simulink model "Ammonia_Model"  (R2023a)
settings: Solver=FixedStepAuto  StartTime=0.0  StopTime=Z  FixedStep=1/24  RelTol=1e-3
values from neighbouring files (symbols this model uses):
  c_eh = 0.85    [Model_Parameters.m]
  cc_AH2_l = 0.6    [Model_Parameters.m]
  cc_AH2_r = 0.75    [Model_Parameters.m]
  cc_AH2_z = 0.65    [Model_Parameters.m]
  cc_e = -0.85    [Model_Parameters.m]
  id_l_A = id_l*id_frac_A    (= 0.0480384)    [Model_Parameters.m]
  id_r_A = id_r*id_frac_A    (= 0.1479168)    [Model_Parameters.m]
  id_z_A = id_z*id_frac_A    (= 0.114048)    [Model_Parameters.m]
  R_ammonia = 0.025    [Model_Parameters.m]
  R_H2 = 0.05    [Model_Parameters.m]
  R_lh = 0.025    [Model_Parameters.m]
  R_ng = 0.025    [Model_Parameters.m]
  S_a_l = 0.3    [Model_Parameters.m]
  S_a_r = 0.2    [Model_Parameters.m]
  S_a_z = 0.25    [Model_Parameters.m]
libraries: fl_lib x72, nesl_utility x50, ee_lib x27
(part 1 of 2)
settings Model: Creator=pienv  LastModifiedBy=pienv

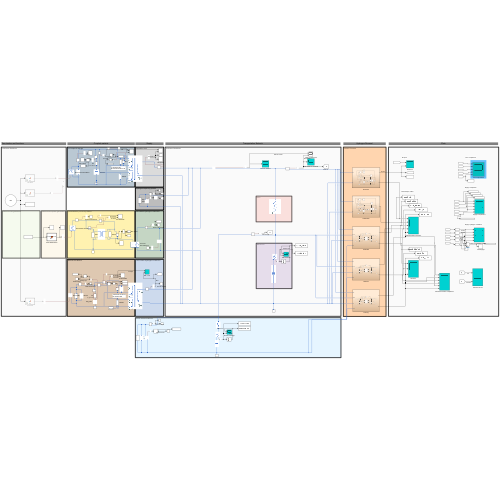
[thumbnail: Simulink's stored preview of the top-level diagram]
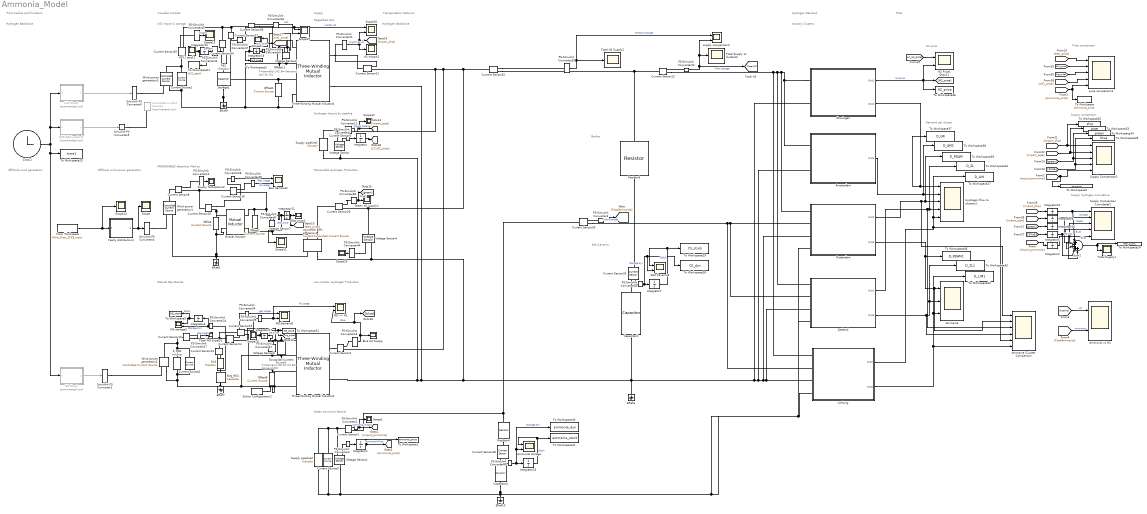
== system Ammonia_Model ==
  note: Supply hydrogen cumulative
  note: T=demand NG for H2
      | B= demand NG
  note: Demand per cluster
  note: LH2 Import & storage
  note: Plots
  note: Salt Caverns
  note: Offshore wind generation
  note: Price comparison
  note: Broker
  note: Coupled markets
  note: Natural Gas Market
  note: (RENEWABLE) electricity Market
  note: Hydrogen Backbone
  note: Hydrogen Import by pipeline
  note: Offshore wind power generation
  note: Green ammonia Market
  note: Time tracker and functions
  note: T=demand LH2
      | B= demand LH2 for H2
  note: H2 price
  note: Supply
  note: Hydrogen Demand
  note: Regasified LH2
  note: Renewable Hydrogen Production
  note: Transportation Network
  note: Hydrogen Backbone
  note: Industry Clusters
  note: Supply comparison
  note: Low-Carbon Hydrogen Production
  Ammonia : Scope  NumInputPorts=3
  Ammonia CLuster Comparison : Scope  NumInputPorts=6
  Ammonia storage : Scope  NumInputPorts=2
  Ammonia vs H2 : Scope  NumInputPorts=2
  Amsterdam : Subsystem
  Blue H2 Supply : Scope
  Capacitor3 : fl_lib/Electrical/Electrical Elements/Capacitor  c=C_sc F  r=0 Ohm  g=0 1/Ohm  i_specify=on  i_priority=None  i=0.1 A  i_nominal_specify=off  i_nominal_unit=A  i_nominal_value=0.1  v_specify=off  v_priority=None  v=0 V  v_nominal_specify=off  v_nominal_unit=V  v_nominal_value=1  vc_specify=off  vc_priority=High  vc=0 V  vc_nominal_specify=off  vc_nominal_unit=V  vc_nominal_value=1
  Capacitor4 : fl_lib/Electrical/Electrical Elements/Capacitor  c=C_ammonia F  r=0 Ohm  g=0 1/Ohm  i_specify=on  i_priority=None  i=0.1 A  i_nominal_specify=off  i_nominal_unit=A  i_nominal_value=0.1  v_specify=off  v_priority=None  v=0 V  v_nominal_specify=off  v_nominal_unit=V  v_nominal_value=1  vc_specify=off  vc_priority=High  vc=0 V  vc_nominal_specify=off  vc_nominal_unit=V  vc_nominal_value=1
  Clock2 : Clock
      settings: Decimation=24
  Controlled Current Source1 : fl_lib/Electrical/Electrical Sources/Controlled Current Source  Commented=on
  Current Sensor{1,3,8..16,26,29,32..39} (21 alike) : fl_lib/Electrical/Electrical Sensors/Current Sensor
  Current Source1 : ee_lib/Sources/Current Source  dc_current=I_LH2 A  ac_current=0 A  ac_shift=0 rad  ac_frequency=60 Hz  noise_mode=ee.enum.sources.noise.Disabled  PSD=0 A^2/Hz  sample_time=1e-3 s  repeatability=ee.enum.sources.repeatability.NotRepeatable  user_seed=0  auto_seed=3890346746  i_specify=off  i_priority=None  i=0 A  i_nominal_specify=off  i_nominal_unit=A  i_nominal_value=1  v_specify=off  v_priority=None  v=0 V  v_nominal_specify=off  v_nominal_unit=V  v_nominal_value=1
  Current Source2 : ee_lib/Sources/Current Source  dc_current=v_sng A  ac_current=0 A  ac_shift=0 rad  ac_frequency=60 Hz  noise_mode=ee.enum.sources.noise.Disabled  PSD=0 A^2/Hz  sample_time=1e-3 s  repeatability=ee.enum.sources.repeatability.NotRepeatable  user_seed=0  auto_seed=545404223  i_specify=off  i_priority=None  i=0 A  i_nominal_specify=off  i_nominal_unit=A  i_nominal_value=1  v_specify=off  v_priority=None  v=0 V  v_nominal_specify=off  v_nominal_unit=V  v_nominal_value=1
  Current Source3 : ee_lib/Sources/Current Source  dc_current=I_ammonia A  ac_current=0 A  ac_shift=0 rad  ac_frequency=60 Hz  noise_mode=ee.enum.sources.noise.Disabled  PSD=0 A^2/Hz  sample_time=1e-3 s  repeatability=ee.enum.sources.repeatability.NotRepeatable  user_seed=0  auto_seed=3922919431  i_specify=off  i_priority=None  i=0 A  i_nominal_specify=off  i_nominal_unit=A  i_nominal_value=1  v_specify=off  v_priority=None  v=0 V  v_nominal_specify=off  v_nominal_unit=V  v_nominal_value=1
  ERef{6..10} (5 alike) : fl_lib/Electrical/Electrical Elements/Electrical Reference
  Elec demand2 : Scope  NumInputPorts=2
  Elec price1 : Scope
  From Workspace : FromWorkspace  VariableName=Wind_Distr_2019_input  OutDataTypeStr=double
  Green H2 supply2 : Scope
  Groningen : Subsystem
  H2 Import2 : Scope
  H2 Price1 : Scope  NumInputPorts=2
  H2(L) stock2 : Scope
  Hydrogen flow to clusters1 : Scope  NumInputPorts=5
  Integrator{,1..2,5..8,10..11,13,17..18,22..23} (14 alike) : Integrator
  LH2 Shock : MATLAB Function  Commented=on  TreatAsAtomicUnit=on
  Limburg : Subsystem
  MATLAB Function2 : MATLAB Function  Commented=on  TreatAsAtomicUnit=on
  Mutual Inductor : fl_lib/Electrical/Electrical Elements/Mutual Inductor  L1=L_eh H  L2=L_e H  k=cc_e  i1_specify=off  i1_priority=High  i1=0 A  i1_nominal_specify=off  i1_nominal_unit=A  i1_nominal_value=1  i2_specify=off  i2_priority=High  i2=0 A  i2_nominal_specify=off  i2_nominal_unit=A  i2_nominal_value=1  v1_specify=off  v1_priority=None  v1=0 V  v1_nominal_specify=off  v1_nominal_unit=V  v1_nominal_value=1  v2_specify=off  v2_priority=None  v2=0 V  v2_nominal_specify=off  v2_nominal_unit=V  v2_nominal_value=1
      settings: InternalSimscapePortConfiguration="{\"Bottom\":[],\"Left\":[{\"id\":\"p1\",\"label\":\"1+\",\"type\":\"foundation.electrical.electrical\"},{\"id\":\"n1\",\"label\":\"1-\",\"type\":\"foundation.electrical.electrical\"}],\"Right\":[{\"id\":\"p2\",\"label\":\"2+\",\"type\":\"foundation.electrical.electrical\"},{\"id\":\"n2\",\"label\":\"2-\",\"type\":\"foundation.electrical.electrical\"}],\"Top\":[]}"
  NG --> H1 : Scope  NumInputPorts=2
  NG Shock : MATLAB Function  Commented=on  TreatAsAtomicUnit=on
  NG demand2 : Scope  NumInputPorts=2
  NG storage2 : Scope  NumInputPorts=2
  Offset1 : ee_lib/Sources/Current Source  dc_current=id_lh2h A  ac_current=0 A  ac_shift=0 rad  ac_frequency=0 Hz  noise_mode=0  PSD=0 A^2/Hz  sample_time=1e-3 s  repeatability=1  user_seed=0  auto_seed=2348838240  i_specify=off  i_priority=None  i=0 A  i_nominal_specify=off  i_nominal_unit=A  i_nominal_value=1  v_specify=off  v_priority=None  v=0 V  v_nominal_specify=off  v_nominal_unit=V  v_nominal_value=1
  Offset11 : ee_lib/Sources/Current Source  dc_current=id_lh2 A  ac_current=0 A  ac_shift=0 rad  ac_frequency=0 Hz  noise_mode=0  PSD=0 A^2/Hz  sample_time=1e-3 s  repeatability=1  user_seed=0  auto_seed=4112460543  i_specify=off  i_priority=None  i=0 A  i_nominal_specify=off  i_nominal_unit=A  i_nominal_value=1  v_specify=off  v_priority=None  v=0 V  v_nominal_specify=off  v_nominal_unit=V  v_nominal_value=1
  Offset2 : ee_lib/Sources/Current Source  dc_current=id_eh A  ac_current=0 A  ac_shift=0 rad  ac_frequency=0 Hz  noise_mode=0  PSD=0 A^2/Hz  sample_time=1e-3 s  repeatability=1  user_seed=0  auto_seed=4144164703  i_specify=off  i_priority=None  i=0 A  i_nominal_specify=off  i_nominal_unit=A  i_nominal_value=1  v_specify=off  v_priority=None  v=0 V  v_nominal_specify=off  v_nominal_unit=V  v_nominal_value=1
  Offset9 : ee_lib/Sources/Current Source  dc_current=id_ngh A  ac_current=0 A  ac_shift=0 rad  ac_frequency=0 Hz  noise_mode=0  PSD=0 A^2/Hz  sample_time=1e-3 s  repeatability=1  user_seed=0  auto_seed=676943032  i_specify=off  i_priority=None  i=0 A  i_nominal_specify=off  i_nominal_unit=A  i_nominal_value=1  v_specify=off  v_priority=None  v=0 V  v_nominal_specify=off  v_nominal_unit=V  v_nominal_value=1
  Offst3 : ee_lib/Sources/Current Source  dc_current=id_e A  ac_current=0 A  ac_shift=0 rad  ac_frequency=0 Hz  noise_mode=0  PSD=0 A^2/Hz  sample_time=1e-3 s  repeatability=1  user_seed=0  auto_seed=4168664255  i_specify=off  i_priority=None  i=0 A  i_nominal_specify=off  i_nominal_unit=A  i_nominal_value=1  v_specify=off  v_priority=None  v=0 V  v_nominal_specify=off  v_nominal_unit=V  v_nominal_value=1
  PS-Simulink Converter{1..3,8..9,11..12,16,21..22,24,27..29,34..35,37..42,44..45,49} (25 alike) : nesl_utility/PS-Simulink Converter  PhysicalDomain=network_engine_domain  SubClassName=ps_output  LeftPortType=input  RightPortType=output  PseudoPeriodic=off  Frequencies=[]  VectorFormat=1-D array  Unit=1  AffineConversion=off
  PS-Simulink Converter46 : nesl_utility/PS-Simulink Converter  PhysicalDomain=network_engine_domain  SubClassName=ps_output  LeftPortType=input  RightPortType=output  PseudoPeriodic=off  Frequencies=[]  VectorFormat=inherit  Unit=inherit  AffineConversion=off
  PS-Simulink Converter47 : nesl_utility/PS-Simulink Converter  PhysicalDomain=network_engine_domain  SubClassName=ps_output  LeftPortType=input  RightPortType=output  PseudoPeriodic=off  Frequencies=[]  VectorFormat=inherit  Unit=inherit  AffineConversion=off
  Resistor3 : fl_lib/Electrical/Electrical Elements/Resistor  R=R_H2 Ohm  i_specify=off  i_priority=None  i=0 A  i_nominal_specify=off  i_nominal_unit=A  i_nominal_value=1  v_specify=off  v_priority=None  v=0 V  v_nominal_specify=off  v_nominal_unit=V  v_nominal_value=1
  Resistor4 : fl_lib/Electrical/Electrical Elements/Resistor  R=R_ammonia Ohm  i_specify=off  i_priority=None  i=0 A  i_nominal_specify=off  i_nominal_unit=A  i_nominal_value=1  v_specify=off  v_priority=None  v=0 V  v_nominal_specify=off  v_nominal_unit=V  v_nominal_value=1
  Rotterdam : Subsystem
  S_NG2 : ee_lib/Passive/Inductor  l=L_sng H  enable_L_tol=ee.enum.toleranceApplication.none  L_tol=20  tol_distribution=ee.enum.toleranceDistribution.uniform  nSigma=4  r=0 Ohm  g=0 1/Ohm  enable_operating_limits=ee.enum.enable.no  operating_limit_action=ee.enum.passive.reportOpLim.warn  max_working_current=1 A  power_rating=1 W  enable_faults=ee.enum.enable.no  fault_action=simscape.enum.assert.action.none  lambdaPercent=50  k_faulted=0.9999  turnsShort=ee.enum.passive.inductor.turnsShortOption.no  openCct=ee.enum.enable.no  groundShort=ee.enum.passive.inductor.groundShortOption.no  groundShortG=0 1/Ohm  tau_fault=1e-3 s  fault_trigger=ee.enum.faults.faultTrigger.temporal  t_fault=1 s  max_permissible_voltage=100 V  n_fail_on_voltage=1  max_permissible_current=1 A  t_fail_on_current=1 s  i_L_specify=off  i_L_priority=High  i_L=0 A  i_L_nominal_specify=off  i_L_nominal_unit=A  i_L_nominal_value=1
  Salt Caverns3 : Scope  NumInputPorts=2
  Scope{,1,11..14,19..20} (8 alike) : Scope
  Scope15 : Scope  NumInputPorts=2
  Scope16 : Scope  NumInputPorts=2
  Scope17 : Scope  NumInputPorts=2
  Simulink-PS Converter1 : nesl_utility/Simulink-PS Converter  PhysicalDomain=network_engine_domain  SubClassName=ps_input  LeftPortType=input  RightPortType=output  PseudoPeriodic=off  Frequencies=[]  NoiseDistribution=none  NoiseParameters=[]  Unit=1  AffineConversion=off  FilteringAndDerivatives=provide  SimscapeFilterOrder=1  InputFilterTimeConstant=0.001  UdotUserProvided=0
  Simulink-PS Converter4 : nesl_utility/Simulink-PS Converter  PhysicalDomain=network_engine_domain  SubClassName=ps_input  LeftPortType=input  RightPortType=output  PseudoPeriodic=off  Frequencies=[]  NoiseDistribution=none  NoiseParameters=[]  Unit=1  AffineConversion=off  FilteringAndDerivatives=filter  SimscapeFilterOrder=2  InputFilterTimeConstant=0.001  UdotUserProvided=0
  Simulink-PS Converter5 : nesl_utility/Simulink-PS Converter  PhysicalDomain=network_engine_domain  SubClassName=ps_input  LeftPortType=input  RightPortType=output  PseudoPeriodic=off  Frequencies=[]  NoiseDistribution=none  NoiseParameters=[]  Unit=1  AffineConversion=off  FilteringAndDerivatives=provide  SimscapeFilterOrder=1  InputFilterTimeConstant=0.001  UdotUserProvided=0
  Simulink-PS Converter6 : nesl_utility/Simulink-PS Converter  PhysicalDomain=network_engine_domain  SubClassName=ps_input  LeftPortType=input  RightPortType=output  PseudoPeriodic=off  Frequencies=[]  NoiseDistribution=none  NoiseParameters=[]  Unit=1  AffineConversion=off  FilteringAndDerivatives=provide  SimscapeFilterOrder=1  InputFilterTimeConstant=0.001  UdotUserProvided=0
  Sinusoidal Current Source1 : ee_lib/Additional Components/SPICE Sources/Sinusoidal Current Source  IO=id_ng_IO A  IA=id_ng_IA A  FREQ=id_ng_FREQ Hz  TD=id_ng_TD s  DF=0 1/s  Gmin_param=ee.enum.gminParam.yes
      settings: InternalSimscapePortConfiguration="{\"Bottom\":[],\"Left\":[{\"id\":\"p\",\"label\":\"+\",\"type\":\"foundation.electrical.electrical\"}],\"Right\":[{\"id\":\"n\",\"label\":\"-\",\"type\":\"foundation.electrical.electrical\"}],\"Top\":[]}"
  Solver Configuration2 : nesl_utility/Solver Configuration  PhysicalDomain=network_engine_domain  SubClassName=solver  LeftPortType=input  RightPortType=generic  Tones=[]  Harmonics=[]  SimulateNoise=off  Profile=off  UseLocalSampling=off  EnableSwitchedLinearOptims=on  FrequencyDomain=off  UseCCode=off  RelTol=0.001  AbsTol=0.001  MinStep=1e-09  ToWorkspace=off  RevertToSquareIcSolve=off  NumHomotopyIterations=100  PhasorMode=off  PhasorModeNumHarmonics=1  ConsistencySolver=NEWTON_XTOL_AFTER_FTOL  IndexReductionMethod=DerivativeReplacement  DoDC=off  ResidualTolerance=1e-09  ConsistencyTolSource=LOCAL  ConsistencyAbsTol=0.001  ConsistencyRelTol=0.001  ConsistencyTolFactor=0.001  UseLocalSolver=off  LocalSolverChoice=NE_BACKWARD_EULER_ADVANCER  ResolveIndetEquations=on  FunctionEvalNumThread=1  LocalSolverSampleTime=0.001  DoFixedCost=off  MaxNonlinIter=3  MaxModeIter=2  ComputeImpulses=off  ImpulseIterations=2  LinearAlgebra=auto  LinearAlgebraNumThread=0  EquationFormulation=NE_TIME_EF  DelaysMemoryBudget=1024  AutomaticFiltering=off  FilteringTimeConstant=0.0001  PartitionStorageMethod=AS_NEEDED  PartitionMemoryBudget=1024  PartitionMethod=ROBUST
  Storage1 : fl_lib/Electrical/Electrical Elements/Capacitor  c=C_lh F  r=0 Ohm  g=0 1/Ohm  i_specify=off  i_priority=None  i=0 A  i_nominal_specify=off  i_nominal_unit=A  i_nominal_value=1  v_specify=off  v_priority=None  v=0 V  v_nominal_specify=off  v_nominal_unit=V  v_nominal_value=1  vc_specify=off  vc_priority=High  vc=0 V  vc_nominal_specify=off  vc_nominal_unit=V  vc_nominal_value=1
  Strg_NG1 : fl_lib/Electrical/Electrical Elements/Capacitor  c=C_ng F  r=0 Ohm  g=0 1/Ohm  i_specify=off  i_priority=None  i=0 A  i_nominal_specify=off  i_nominal_unit=A  i_nominal_value=1  v_specify=off  v_priority=None  v=0 V  v_nominal_specify=off  v_nominal_unit=V  v_nominal_value=1  vc_specify=off  vc_priority=High  vc=0 V  vc_nominal_specify=off  vc_nominal_unit=V  vc_nominal_value=100
  Sum2 : Sum  Inputs=|+++++
  Supply pipeline1 : ee_lib/Passive/Inductor  l=L_i H  enable_L_tol=ee.enum.toleranceApplication.none  L_tol=20  tol_distribution=ee.enum.toleranceDistribution.uniform  nSigma=4  r=0 Ohm  g=0 1/Ohm  enable_operating_limits=ee.enum.enable.no  operating_limit_action=ee.enum.passive.reportOpLim.warn  max_working_current=1 A  power_rating=1 W  enable_faults=ee.enum.enable.no  fault_action=simscape.enum.assert.action.none  lambdaPercent=50  k_faulted=0.9999  turnsShort=ee.enum.passive.inductor.turnsShortOption.no  openCct=ee.enum.enable.no  groundShort=ee.enum.passive.inductor.groundShortOption.no  groundShortG=0 1/Ohm  tau_fault=1e-3 s  fault_trigger=ee.enum.faults.faultTrigger.temporal  t_fault=1 s  max_permissible_voltage=100 V  n_fail_on_voltage=1  max_permissible_current=1 A  t_fail_on_current=1 s  i_L_specify=off  i_L_priority=High  i_L=0 A  i_L_nominal_specify=off  i_L_nominal_unit=A  i_L_nominal_value=1
  Supply pipeline2 : ee_lib/Passive/Inductor  l=L_ammonia H  enable_L_tol=ee.enum.toleranceApplication.none  L_tol=20  tol_distribution=ee.enum.toleranceDistribution.uniform  nSigma=4  r=0 Ohm  g=0 1/Ohm  enable_operating_limits=ee.enum.enable.no  operating_limit_action=ee.enum.passive.reportOpLim.warn  max_working_current=1 A  power_rating=1 W  enable_faults=ee.enum.enable.no  fault_action=simscape.enum.assert.action.none  lambdaPercent=50  k_faulted=0.9999  turnsShort=ee.enum.passive.inductor.turnsShortOption.no  openCct=ee.enum.enable.no  groundShort=ee.enum.passive.inductor.groundShortOption.no  groundShortG=0 1/Ohm  tau_fault=1e-3 s  fault_trigger=ee.enum.faults.faultTrigger.temporal  t_fault=1 s  max_permissible_voltage=100 V  n_fail_on_voltage=1  max_permissible_current=1 A  t_fail_on_current=1 s  i_L_specify=off  i_L_priority=High  i_L=0 A  i_L_nominal_specify=off  i_L_nominal_unit=A  i_L_nominal_value=1
  Supply Comparison Cumulatief1 : Scope  NumInputPorts=5
  Supply Comparison1 : Scope  NumInputPorts=5
  Supply fluctuations2 : Scope
  Three-Winding Mutual Inductor3 : ee_lib/Passive/Transformers/Three-Winding Mutual Inductor  L1=L_sbh H  L2=L_ngh H  L3=L_ng H  K12=c_ng12  K13=c_ng13  K23=c_ng23  IC_given=1  IC1=0 A  IC2=0 A  IC3=0 A
      settings: LogSimulationData=on  InternalSimscapePortConfiguration="{\"Bottom\":[],\"Left\":[{\"id\":\"p1\",\"label\":\"1+\",\"type\":\"foundation.electrical.electrical\"},{\"id\":\"n1\",\"label\":\"1-\",\"type\":\"foundation.electrical.electrical\"}],\"Right\":[{\"id\":\"p2\",\"label\":\"2+\",\"type\":\"foundation.electrical.electrical\"},{\"id\":\"n2\",\"label\":\"2-\",\"type\":\"foundation.electrical.electrical\"},{\"id\":\"p3\",\"label\":\"3+\",\"type\":\"foundation.electrical.electrical\"},{\"id\":\"n3\",\"label\":\"3-\",\"type\":\"foundation.electrical.electrical\"}],\"Top\":[]}"
  Three-Winding Mutual Inductor4 : ee_lib/Passive/Transformers/Three-Winding Mutual Inductor  L1=L_sih H  L2=L_lh2h H  L3=L_lh2 H  K12=c_lh212  K13=c_lh213  K23=c_lh223  IC_given=1  IC1=0 A  IC2=0 A  IC3=0 A
      settings: LogSimulationData=on  InternalSimscapePortConfiguration="{\"Bottom\":[],\"Left\":[{\"id\":\"p1\",\"label\":\"1+\",\"type\":\"foundation.electrical.electrical\"},{\"id\":\"n1\",\"label\":\"1-\",\"type\":\"foundation.electrical.electrical\"}],\"Right\":[{\"id\":\"p2\",\"label\":\"2+\",\"type\":\"foundation.electrical.electrical\"},{\"id\":\"n2\",\"label\":\"2-\",\"type\":\"foundation.electrical.electrical\"},{\"id\":\"p3\",\"label\":\"3+\",\"type\":\"foundation.electrical.electrical\"},{\"id\":\"n3\",\"label\":\"3-\",\"type\":\"foundation.electrical.electrical\"}],\"Top\":[]}"
  To Workspace : ToWorkspace  VariableName=Ammonia_price  SampleTime=-1
  To Workspace1 : ToWorkspace  VariableName=ammonia_price  SampleTime=-1
  To Workspace17 : ToWorkspace  VariableName=LH2_stock  SampleTime=-1
  To Workspace2 : ToWorkspace  VariableName=ammonia  SampleTime=-1
  To Workspace24 : ToWorkspace  VariableName=total_supply  SampleTime=-1
  To Workspace25 : ToWorkspace  VariableName=time1  SampleTime=-1
  To Workspace26 : ToWorkspace  VariableName=D_ZL  SampleTime=-1
      settings: Save2DSignal=2-D array (concatenate along first dimension)
  To Workspace27 : ToWorkspace  VariableName=D_LIM  SampleTime=-1
      settings: Save2DSignal=2-D array (concatenate along first dimension)
  To Workspace28 : ToWorkspace  VariableName=CS_dyn  SampleTime=-1
      settings: Save2DSignal=2-D array (concatenate along first dimension)
  To Workspace29 : ToWorkspace  VariableName=CS_stock  SampleTime=-1
  To Workspace3 : ToWorkspace  VariableName=LH2_price  SampleTime=-1
  To Workspace31 : ToWorkspace  VariableName=NG_price  SampleTime=-1
      settings: Save2DSignal=2-D array (concatenate along first dimension)
  To Workspace32 : ToWorkspace  VariableName=ship  SampleTime=-1
  To Workspace33 : ToWorkspace  VariableName=pipe  SampleTime=-1
  To Workspace34 : ToWorkspace  VariableName=green  SampleTime=-1
  To Workspace35 : ToWorkspace  VariableName=blue  SampleTime=-1
  To Workspace36 : ToWorkspace  VariableName=H2_price  SampleTime=-1
  To Workspace37 : ToWorkspace  VariableName=D_GR  SampleTime=-1
      settings: Save2DSignal=2-D array (concatenate along first dimension)
  To Workspace38 : ToWorkspace  VariableName=D_AMS  SampleTime=-1
      settings: Save2DSignal=2-D array (concatenate along first dimension)
  To Workspace39 : ToWorkspace  VariableName=D_RDAM  SampleTime=-1
      settings: Save2DSignal=2-D array (concatenate along first dimension)
  To Workspace40 : ToWorkspace  VariableName=ammonia_dyn  SampleTime=-1
      settings: Save2DSignal=2-D array (concatenate along first dimension)
  To Workspace41 : ToWorkspace  VariableName=ammonia_stock  SampleTime=-1
  To Workspace42 : ToWorkspace  VariableName=D_ZL1  SampleTime=-1
      settings: Save2DSignal=2-D array (concatenate along first dimension)
  To Workspace43 : ToWorkspace  VariableName=D_LIM1  SampleTime=-1
      settings: Save2DSignal=2-D array (concatenate along first dimension)
  To Workspace46 : ToWorkspace  VariableName=D_RDAM1  SampleTime=-1
      settings: Save2DSignal=2-D array (concatenate along first dimension)
  To Workspace5 : ToWorkspace  VariableName=NG_stock  SampleTime=-1
  Total H2 Supply2 : Scope
  Total NG Supply1 : Scope
  Total Supply to clusters2 : Scope
  Total Supply1 : Scope
  Voltage Sensor{,1..4,7} (6 alike) : fl_lib/Electrical/Electrical Sensors/Voltage Sensor
  Wind power generation1 : fl_lib/Electrical/Electrical Sources/Controlled Current Source
  Wind power generation2 : fl_lib/Electrical/Electrical Sources/Controlled Current Source
  Wind power generation3 : fl_lib/Electrical/Electrical Sources/Controlled Current Source
  Yearly distribution4 : MATLAB Function  TreatAsAtomicUnit=on
  Zeeland : Subsystem
  conversie 85% efficiency1 : fl_lib/Electrical/Electrical Sources/Current-Controlled Current Source  K=c_eh  i1_specify=off  i1_priority=None  i1=0 A  i1_nominal_specify=off  i1_nominal_unit=A  i1_nominal_value=1  i2_specify=off  i2_priority=None  i2=0 A  i2_nominal_specify=off  i2_nominal_unit=A  i2_nominal_value=1
      settings: InternalSimscapePortConfiguration="{\"Bottom\":[],\"Left\":[{\"id\":\"p1\",\"label\":\"+\",\"type\":\"foundation.electrical.electrical\"},{\"id\":\"head\",\"label\":\"\",\"type\":\"foundation.electrical.electrical\"}],\"Right\":[{\"id\":\"n1\",\"label\":\"-\",\"type\":\"foundation.electrical.electrical\"},{\"id\":\"tail\",\"label\":\"\",\"type\":\"foundation.electrical.electrical\"}],\"Top\":[]}"
  frc1 : fl_lib/Electrical/Electrical Elements/Resistor  R=R_lh Ohm  i_specify=off  i_priority=High  i=0 A  i_nominal_specify=off  i_nominal_unit=A  i_nominal_value=1  v_specify=off  v_priority=High  v=0 V  v_nominal_specify=off  v_nominal_unit=V  v_nominal_value=1
      settings: AttributesFormatString=%<R> %<R_unit>
  frc3 : fl_lib/Electrical/Electrical Elements/Resistor  R=R_ng Ohm  i_specify=off  i_priority=High  i=0 A  i_nominal_specify=off  i_nominal_unit=A  i_nominal_value=1  v_specify=off  v_priority=High  v=0 V  v_nominal_specify=off  v_nominal_unit=V  v_nominal_value=1
      settings: AttributesFormatString=%<R> %<R_unit>
  price comparison2 : Scope  NumInputPorts=5
  supply comparison2 : Scope  NumInputPorts=2
  wires:
  [import_pipe] -> To Workspace33/1, Supply Comparison1/2
  Clock2/1 -> LH2 Shock/1(X), MATLAB Function2/1(X), NG Shock/1(X), To Workspace25/1
  PS-Simulink Converter45/1 -> Scope13/1  "Import"
  Integrator11/1 -> [elec_price], Elec price1/1  "elec price"
  MATLAB Function2/1(y) -> Simulink-PS Converter5/1
  [blue] -> Integrator5/1
  Integrator6/1 -> To Workspace5/1, NG storage2/1  "Stock"
  PS-Simulink Converter47/1 -> Scope16/1, Scope15/1  "LH2 for H2"
  PS-Simulink Converter44/1 -> Scope19/1
  PS-Simulink Converter12/1 -> Supply fluctuations2/1
  [LH2_price] -> price comparison2/4
  PS-Simulink Converter1/1 -> Scope1/1, [import_ammonia]  "Ammonia import"
  Integrator1/1 -> To Workspace1/1, [ammonia_price]  "Ammonia Price"
  PS-Simulink Converter16/1 -> [blue], NG --> H1/2, Blue H2 Supply/1  "Blue"
  PS-Simulink Converter8/1 -> Integrator/1
  PS-Simulink Converter22/1 -> [TotalH2], Total Supply to clusters2/1, supply comparison2/2  "With storage"
  PS-Simulink Converter2/1 -> Integrator1/1
  PS-Simulink Converter11/1 -> Scope12/1, [import_pipe]  "import pipeline"
  [blue] -> To Workspace35/1, Supply Comparison1/4
  [LC_H2_price] -> H2 Price1/1
  PS-Simulink Converter38/1 -> [green], Green H2 supply2/1  "Green"
  Groningen/1(Out1) -> H2 Price1/2, To Workspace36/1, [H2_price]  "H2 price"
  Sum2/1 -> Total Supply1/1, To Workspace24/1
  NG Shock/1(y) -> Simulink-PS Converter1/1
  PS-Simulink Converter37/1 -> Integrator17/1
  [green] -> Integrator10/1
  [elec_price] -> price comparison2/1
  PS-Simulink Converter41/1 -> Scope11/1, Integrator11/1
  Integrator23/1 -> Ammonia storage/1, To Workspace41/1  "Stock"
  PS-Simulink Converter34/1 -> NG demand2/1  "gas Usage"
  PS-Simulink Converter35/1 -> supply comparison2/1, Total H2 Supply2/1  "Without storage"
  PS-Simulink Converter9/1 -> Integrator18/1
  [import_pipe] -> Integrator8/1
  Groningen/2(Out2) -> Hydrogen flow to clusters1/1, To Workspace37/1
  Integrator13/1 -> To Workspace17/1, H2(L) stock2/1
  Yearly distribution4/1(current) -> Scope/1, Simulink-PS Converter4/1
  [import_ship] -> To Workspace32/1, Supply Comparison1/1
  Integrator5/1 -> Supply Comparison Cumulatief1/4, Sum2/4  "Blue"
  PS-Simulink Converter27/1 -> Total NG Supply1/1  "NG supply"
  Integrator/1 -> [LC_H2_price]
  Integrator10/1 -> Supply Comparison Cumulatief1/3, Sum2/5, Sum2/3  "Green"
  PS-Simulink Converter24/1 -> Integrator6/1, NG storage2/2  "Storage dyn"
  [ammonia_price] -> To Workspace/1, price comparison2/5
  LH2 Shock/1(y) -> Simulink-PS Converter6/1
  PS-Simulink Converter28/1 -> Elec demand2/1  "Elec Usage"
  Integrator17/1 -> [ng_price], To Workspace31/1, Scope20/1  "NG price"
  Integrator22/1 -> Supply Comparison Cumulatief1/1, Sum2/1  "H2 ship"
  PS-Simulink Converter49/1 -> To Workspace40/1, Ammonia storage/2, Integrator23/1  "Storage dyn"
  [H2_price] -> price comparison2/2
  Integrator18/1 -> To Workspace3/1, Scope17/1, [LH2_price]  "LH2 price"
  [green] -> To Workspace34/1, Supply Comparison1/3
  PS-Simulink Converter42/1 -> Integrator13/1  "Import"
  [ng_price] -> price comparison2/3
  PS-Simulink Converter46/1 -> Scope15/2  "LH2"
  Amsterdam/1(Out2) -> To Workspace38/1, Hydrogen flow to clusters1/2
  Integrator7/1 -> To Workspace29/1, Salt Caverns3/1  "Stock"
  PS-Simulink Converter21/1 -> Scope16/2, [import_ship], H2 Import2/1  "Import H2 (L)"
  PS-Simulink Converter40/1 -> To Workspace28/1, Salt Caverns3/2, Integrator7/1  "Storage dyn"
  PS-Simulink Converter29/1 -> NG --> H1/1, NG demand2/2  "H2 usage"
  PS-Simulink Converter39/1 -> Elec demand2/2  "H2 usage"
  Integrator8/1 -> Supply Comparison Cumulatief1/2, Sum2/2  "H2 pipe"
  [import_ship] -> Integrator22/1
  From Workspace/1 -> Scope14/1, Yearly distribution4/1(wind_distr)
  Rotterdam/1(Out2) -> Ammonia CLuster Comparison/1, Hydrogen flow to clusters1/3, To Workspace39/1
  Zeeland/2(Out5) -> Ammonia CLuster Comparison/4, To Workspace42/1, Ammonia/2
  Rotterdam/2(Out5) -> Ammonia CLuster Comparison/2, Ammonia/1, To Workspace46/1
  Limburg/2(Out5) -> Ammonia/3, To Workspace43/1, Ammonia CLuster Comparison/6
  [TotalAmmonia] -> Ammonia vs H2/2  "Ammonia"
  Limburg/1(Out2) -> Ammonia CLuster Comparison/5, To Workspace27/1, Hydrogen flow to clusters1/5
  Zeeland/1(Out2) -> Ammonia CLuster Comparison/3, Hydrogen flow to clusters1/4, To Workspace26/1
  [TotalH2] -> Ammonia vs H2/1  "H2"
  PS-Simulink Converter3/1 -> [TotalAmmonia]  "With storage"
  [import_ammonia] -> Integrator2/1
  Integrator2/1 -> Supply Comparison Cumulatief1/5  "Blue"
  [import_ammonia] -> To Workspace2/1, Supply Comparison1/5
  connections:
  Current Source1/RConn1 -- Wind power generation3/RConn2 -- Offset1/LConn1 -- Three-Winding Mutual Inductor4/RConn1 -- Offset11/LConn1 -- Voltage Sensor2/LConn1 -- Three-Winding Mutual Inductor4/RConn3 -- Storage1/LConn1 -- ERef9/LConn1
  Current Sensor37/LConn1 -- Current Sensor36/LConn1 -- Current Sensor35/RConn2 -- Current Sensor34/LConn1
  Three-Winding Mutual Inductor3/RConn2 -- Offset9/RConn1 -- Current Sensor15/RConn2
  Voltage Sensor7/LConn1 -- conversie 85% efficiency1/LConn1 -- Mutual Inductor/LConn1 -- Offset2/LConn1
  ERef7/LConn1 -- S_NG2/LConn1 -- Current Source2/RConn1 -- Wind power generation2/RConn2 -- Strg_NG1/LConn1 -- Three-Winding Mutual Inductor3/RConn1 -- Offset9/LConn1 -- Solver Configuration2/RConn1 -- Three-Winding Mutual Inductor3/RConn3 -- Sinusoidal Current Source1/RConn1 -- Voltage Sensor3/LConn1
  Current Sensor32/LConn1 -- Voltage Sensor4/LConn1 -- Current Sensor29/RConn2 -- Current Sensor9/RConn2 -- Current Sensor11/RConn2 -- Current Sensor3/RConn2
  Groningen/LConn1 -- Rotterdam/LConn1 -- Zeeland/LConn1 -- Limburg/LConn1 -- Current Sensor12/RConn2 -- Amsterdam/LConn1
  Resistor4/RConn1 -- Current Sensor39/LConn1 -- Current Sensor1/RConn2
  Wind power generation2/LConn1 -- Current Source2/LConn1 -- S_NG2/RConn1 -- Current Sensor10/LConn1
  Three-Winding Mutual Inductor4/RConn2 -- Current Sensor37/RConn2 -- Offset1/RConn1
  Voltage Sensor1/LConn1 -- Current Source3/RConn1 -- Supply pipeline2/LConn1 -- ERef10/LConn1 -- Capacitor4/LConn1 -- Limburg/LConn4 -- Zeeland/LConn4 -- Rotterdam/LConn4
  Current Sensor26/LConn1 -- Current Sensor8/RConn2 -- Current Sensor16/LConn1
  Rotterdam/LConn3 -- Amsterdam/LConn2 -- Groningen/LConn2 -- conversie 85% efficiency1/RConn2 -- Voltage Sensor4/RConn2 -- Three-Winding Mutual Inductor3/LConn1 -- Supply pipeline1/LConn1 -- Voltage Sensor/LConn1 -- Three-Winding Mutual Inductor4/LConn1 -- ERef6/LConn1 -- Capacitor3/LConn1 -- Limburg/LConn3 -- Zeeland/LConn3
  Supply pipeline1/RConn1 -- Voltage Sensor/RConn2 -- Current Sensor9/LConn1
  Limburg/LConn2 -- Current Sensor39/RConn2 -- Zeeland/LConn2 -- Rotterdam/LConn2
  Current Sensor14/LConn1 -- Current Sensor10/RConn2 -- Current Sensor13/LConn1 -- Current Sensor15/LConn1
  conversie 85% efficiency1/RConn1 -- Mutual Inductor/RConn1 -- Offst3/LConn1 -- ERef8/LConn1 -- Wind power generation1/RConn2
  Mutual Inductor/RConn2 -- Offst3/RConn1 -- Current Sensor26/RConn2
  Current Sensor35/LConn1 -- Wind power generation3/LConn1 -- Current Source1/LConn1
  Current Sensor1/LConn1 -- Voltage Sensor1/RConn2 -- Current Source3/LConn1 -- Supply pipeline2/RConn1
  Mutual Inductor/LConn2 -- Offset2/RConn1 -- Voltage Sensor7/RConn2 -- Current Sensor16/RConn2
  Current Sensor36/RConn2 -- Voltage Sensor2/RConn2 -- Three-Winding Mutual Inductor4/RConn4 -- Offset11/RConn1
  Current Sensor14/RConn2 -- Voltage Sensor3/RConn2 -- Sinusoidal Current Source1/LConn1 -- Three-Winding Mutual Inductor3/RConn4
  Current Sensor32/RConn2 -- Current Sensor12/LConn1 -- Resistor3/RConn1
  PS-Simulink Converter42/LConn1 -- Current Sensor34/RConn1
  Current Sensor13/RConn1 -- PS-Simulink Converter24/LConn1
  Simulink-PS Converter1/RConn1 -- Wind power generation2/RConn1
  Three-Winding Mutual Inductor4/LConn2 -- Current Sensor11/LConn1
  PS-Simulink Converter37/LConn1 -- Voltage Sensor3/RConn1
  PS-Simulink Converter41/LConn1 -- Voltage Sensor7/RConn1
  PS-Simulink Converter27/LConn1 -- Current Sensor10/RConn1
  Storage1/RConn1 -- frc1/LConn1
  PS-Simulink Converter22/LConn1 -- Current Sensor12/RConn1
  Resistor3/LConn1 -- Current Sensor33/LConn1
  Simulink-PS Converter4/RConn1 -- Wind power generation1/RConn1
  PS-Simulink Converter9/LConn1 -- Voltage Sensor2/RConn1
  Current Sensor26/RConn1 -- PS-Simulink Converter28/LConn1
  Simulink-PS Converter5/RConn1 -- Controlled Current Source1/RConn1
  Current Sensor8/LConn1 -- Wind power generation1/LConn1
  PS-Simulink Converter21/LConn1 -- Current Sensor11/RConn1
  PS-Simulink Converter47/LConn1 -- Current Sensor37/RConn1
  Current Sensor29/LConn1 -- conversie 85% efficiency1/LConn2
  PS-Simulink Converter1/LConn1 -- Current Sensor1/RConn1
  PS-Simulink Converter45/LConn1 -- Current Sensor35/RConn1
  PS-Simulink Converter49/LConn1 -- Current Sensor38/RConn1
  PS-Simulink Converter39/LConn1 -- Current Sensor16/RConn1
  PS-Simulink Converter40/LConn1 -- Current Sensor33/RConn1
  PS-Simulink Converter29/LConn1 -- Current Sensor15/RConn1
  PS-Simulink Converter44/LConn1 -- Voltage Sensor4/RConn1
  Current Sensor38/RConn2 -- Capacitor4/RConn1
  PS-Simulink Converter2/LConn1 -- Voltage Sensor1/RConn1
  PS-Simulink Converter34/LConn1 -- Current Sensor14/RConn1
  PS-Simulink Converter46/LConn1 -- Current Sensor36/RConn1
  PS-Simulink Converter8/LConn1 -- Voltage Sensor/RConn1
  Three-Winding Mutual Inductor3/LConn2 -- Current Sensor3/LConn1
  PS-Simulink Converter16/LConn1 -- Current Sensor3/RConn1
  Current Sensor13/RConn2 -- frc3/RConn1
  frc1/RConn1 -- Current Sensor34/RConn2
  PS-Simulink Converter11/LConn1 -- Current Sensor9/RConn1
  Current Sensor32/RConn1 -- PS-Simulink Converter35/LConn1
  Current Sensor33/RConn2 -- Capacitor3/RConn1
  PS-Simulink Converter38/LConn1 -- Current Sensor29/RConn1
  Current Sensor8/RConn1 -- PS-Simulink Converter12/LConn1
  Resistor4/LConn1 -- Current Sensor38/LConn1
  frc3/LConn1 -- Strg_NG1/RConn1
  Simulink-PS Converter6/RConn1 -- Wind power generation3/RConn1
  PS-Simulink Converter3/LConn1 -- Current Sensor39/RConn1

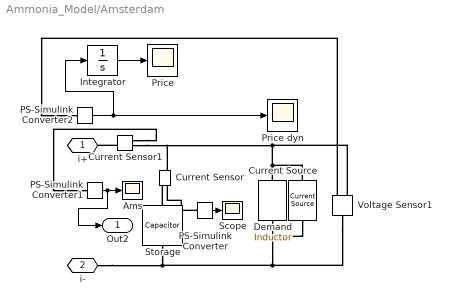
== system Ammonia_Model/Amsterdam ==
  Ams : Scope
  Current Sensor : fl_lib/Electrical/Electrical Sensors/Current Sensor
  Current Sensor1 : fl_lib/Electrical/Electrical Sensors/Current Sensor
  Current Source : ee_lib/Sources/Current Source  dc_current=id_a A  ac_current=0 A  ac_shift=0 rad  ac_frequency=0 Hz  noise_mode=ee.enum.sources.noise.Disabled  PSD=0 A^2/Hz  sample_time=1e-3 s  repeatability=ee.enum.sources.repeatability.NotRepeatable  user_seed=0  auto_seed=3499211588  i_specify=off  i_priority=None  i=0 A  i_nominal_specify=off  i_nominal_unit=A  i_nominal_value=1  v_specify=off  v_priority=None  v=0 V  v_nominal_specify=off  v_nominal_unit=V  v_nominal_value=1
  Demand : ee_lib/Passive/Inductor  l=L_a H  enable_L_tol=0  L_tol=20  tol_distribution=1  nSigma=4  r=0 Ohm  g=0 1/Ohm  enable_operating_limits=0  operating_limit_action=2  max_working_current=1 A  power_rating=1 W  enable_faults=ee.enum.enable.no  fault_action=simscape.enum.assert.action.none  lambdaPercent=50  k_faulted=0.9999  turnsShort=0  openCct=0  groundShort=0  groundShortG=0 1/Ohm  tau_fault=1e-3 s  fault_trigger=ee.enum.faults.faultTrigger.temporal  t_fault=1 s  max_permissible_voltage=100 V  n_fail_on_voltage=1  max_permissible_current=1 A  t_fail_on_current=1 s  i_L_specify=off  i_L_priority=High  i_L=0 A  i_L_nominal_specify=off  i_L_nominal_unit=A  i_L_nominal_value=1
  Integrator : Integrator
  PS-Simulink Converter : nesl_utility/PS-Simulink Converter  PhysicalDomain=network_engine_domain  SubClassName=ps_output  LeftPortType=input  RightPortType=output  PseudoPeriodic=off  Frequencies=[]  VectorFormat=inherit  Unit=inherit  AffineConversion=off
  PS-Simulink Converter1 : nesl_utility/PS-Simulink Converter  PhysicalDomain=network_engine_domain  SubClassName=ps_output  LeftPortType=input  RightPortType=output  PseudoPeriodic=off  Frequencies=[]  VectorFormat=inherit  Unit=inherit  AffineConversion=off
  PS-Simulink Converter2 : nesl_utility/PS-Simulink Converter  PhysicalDomain=network_engine_domain  SubClassName=ps_output  LeftPortType=input  RightPortType=output  PseudoPeriodic=off  Frequencies=[]  VectorFormat=inherit  Unit=inherit  AffineConversion=off
  "Price " : Scope
  Price dyn : Scope
  Scope : Scope
  Storage : fl_lib/Electrical/Electrical Elements/Capacitor  c=C_a F  r=0 Ohm  g=0 1/Ohm  i_specify=off  i_priority=None  i=0 A  i_nominal_specify=off  i_nominal_unit=A  i_nominal_value=1  v_specify=off  v_priority=None  v=0 V  v_nominal_specify=off  v_nominal_unit=V  v_nominal_value=1  vc_specify=off  vc_priority=High  vc=0 V  vc_nominal_specify=off  vc_nominal_unit=V  vc_nominal_value=1
  Voltage Sensor1 : fl_lib/Electrical/Electrical Sensors/Voltage Sensor
  "i+ " : PMIOPort  Tag=PMCPort  Side=Left
  i- : PMIOPort  Tag=PMCPort  Port=2  Side=Left
  Out2 : Outport
  wires:
  PS-Simulink Converter1/1 -> Out2/1, Ams/1
  PS-Simulink Converter/1 -> Scope/1
  Integrator/1 -> "Price "/1
  PS-Simulink Converter2/1 -> Integrator/1, Price dyn/1
  connections:
  Current Source/LConn1 -- Demand/LConn1 -- i-/RConn1 -- Storage/LConn1 -- Voltage Sensor1/LConn1
  Demand/RConn1 -- Current Source/RConn1 -- Current Sensor/LConn1 -- Current Sensor1/RConn2 -- Voltage Sensor1/RConn2
  Voltage Sensor1/RConn1 -- PS-Simulink Converter2/LConn1
  PS-Simulink Converter/LConn1 -- Current Sensor/RConn1
  Current Sensor1/RConn1 -- PS-Simulink Converter1/LConn1
  Current Sensor1/LConn1 -- "i+ "/RConn1
  Storage/RConn1 -- Current Sensor/RConn2

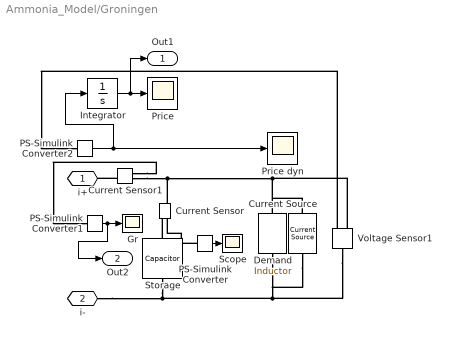
== system Ammonia_Model/Groningen ==
  Current Sensor : fl_lib/Electrical/Electrical Sensors/Current Sensor
  Current Sensor1 : fl_lib/Electrical/Electrical Sensors/Current Sensor
  Current Source : ee_lib/Sources/Current Source  dc_current=id_g A  ac_current=0 A  ac_shift=0 rad  ac_frequency=0 Hz  noise_mode=ee.enum.sources.noise.Disabled  PSD=0 A^2/Hz  sample_time=1e-3 s  repeatability=ee.enum.sources.repeatability.NotRepeatable  user_seed=0  auto_seed=2715962282  i_specify=off  i_priority=None  i=0 A  i_nominal_specify=off  i_nominal_unit=A  i_nominal_value=1  v_specify=off  v_priority=None  v=0 V  v_nominal_specify=off  v_nominal_unit=V  v_nominal_value=1
  Demand : ee_lib/Passive/Inductor  l=L_g H  enable_L_tol=0  L_tol=20  tol_distribution=1  nSigma=4  r=0 Ohm  g=0 1/Ohm  enable_operating_limits=0  operating_limit_action=2  max_working_current=1 A  power_rating=1 W  enable_faults=ee.enum.enable.no  fault_action=simscape.enum.assert.action.none  lambdaPercent=50  k_faulted=0.9999  turnsShort=0  openCct=0  groundShort=0  groundShortG=0 1/Ohm  tau_fault=1e-3 s  fault_trigger=ee.enum.faults.faultTrigger.temporal  t_fault=1 s  max_permissible_voltage=100 V  n_fail_on_voltage=1  max_permissible_current=1 A  t_fail_on_current=1 s  i_L_specify=off  i_L_priority=High  i_L=0 A  i_L_nominal_specify=off  i_L_nominal_unit=A  i_L_nominal_value=1
  Gr : Scope
  Integrator : Integrator
  PS-Simulink Converter : nesl_utility/PS-Simulink Converter  PhysicalDomain=network_engine_domain  SubClassName=ps_output  LeftPortType=input  RightPortType=output  PseudoPeriodic=off  Frequencies=[]  VectorFormat=inherit  Unit=inherit  AffineConversion=off
  PS-Simulink Converter1 : nesl_utility/PS-Simulink Converter  PhysicalDomain=network_engine_domain  SubClassName=ps_output  LeftPortType=input  RightPortType=output  PseudoPeriodic=off  Frequencies=[]  VectorFormat=inherit  Unit=inherit  AffineConversion=off
  PS-Simulink Converter2 : nesl_utility/PS-Simulink Converter  PhysicalDomain=network_engine_domain  SubClassName=ps_output  LeftPortType=input  RightPortType=output  PseudoPeriodic=off  Frequencies=[]  VectorFormat=inherit  Unit=inherit  AffineConversion=off
  "Price " : Scope
  Price dyn : Scope
  Scope : Scope
  Storage : fl_lib/Electrical/Electrical Elements/Capacitor  c=C_g F  r=0 Ohm  g=0 1/Ohm  i_specify=off  i_priority=None  i=0 A  i_nominal_specify=off  i_nominal_unit=A  i_nominal_value=1  v_specify=off  v_priority=None  v=0 V  v_nominal_specify=off  v_nominal_unit=V  v_nominal_value=1  vc_specify=off  vc_priority=High  vc=0 V  vc_nominal_specify=off  vc_nominal_unit=V  vc_nominal_value=1
  Voltage Sensor1 : fl_lib/Electrical/Electrical Sensors/Voltage Sensor
  "i+ " : PMIOPort  Tag=PMCPort  Side=Left
  i- : PMIOPort  Tag=PMCPort  Port=2  Side=Left
  Out1 : Outport
  Out2 : Outport  Port=2
  wires:
  PS-Simulink Converter1/1 -> Out2/1, Gr/1
  Integrator/1 -> Out1/1, "Price "/1
  PS-Simulink Converter2/1 -> Integrator/1, Price dyn/1
  PS-Simulink Converter/1 -> Scope/1
  connections:
  Current Sensor/LConn1 -- Demand/RConn1 -- Current Source/RConn1 -- Voltage Sensor1/RConn2 -- Current Sensor1/RConn2
  Storage/LConn1 -- i-/RConn1 -- Demand/LConn1 -- Current Source/LConn1 -- Voltage Sensor1/LConn1
  Storage/RConn1 -- Current Sensor/RConn2
  Current Sensor1/LConn1 -- "i+ "/RConn1
  PS-Simulink Converter/LConn1 -- Current Sensor/RConn1
  Current Sensor1/RConn1 -- PS-Simulink Converter1/LConn1
  Voltage Sensor1/RConn1 -- PS-Simulink Converter2/LConn1

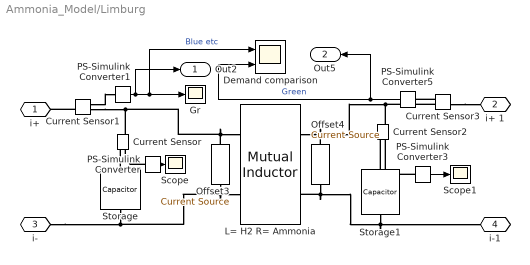
== system Ammonia_Model/Limburg ==
  Current Sensor{,1..3} (4 alike) : fl_lib/Electrical/Electrical Sensors/Current Sensor
  Demand comparison : Scope  NumInputPorts=2
  Gr : Scope
  L= H2 R= Ammonia : ee_lib/Passive/Transformers/Mutual Inductor  L1=L_H2_l H  L2=L_A_l H  k=cc_AH2_l  L_tol=0  enable_L1_tol=ee.enum.toleranceApplication.none  L1_tol_distribution=ee.enum.toleranceDistribution.uniform  L1_nSigma=4  enable_L2_tol=ee.enum.toleranceApplication.none  L2_tol_distribution=ee.enum.toleranceDistribution.uniform  L2_nSigma=4  r=[.001, .001] Ohm  g=[1e-09, 1e-09] 1/Ohm  enable_operating_limits=ee.enum.enable.no  operating_limit_action=ee.enum.passive.reportOpLim.warn  max_working_current=1 A  power_rating=1 W  enable_faults=ee.enum.enable.no  fault_action=simscape.enum.assert.action.none  fault_winding=ee.enum.passive.transformers.faultedWinding.primary  lambdaPercent=50  turnsShort=ee.enum.faults.faultTurnsShort.no  openCct=ee.enum.faults.faultTurnsOpenCkt.no  groundShort=ee.enum.faults.faultTurnsGroundShort.no  groundShortG=0 1/Ohm  tau_fault=1e-3 s  fault_trigger=ee.enum.faults.faultTrigger.temporal  t_fault=1 s  max_permissible_voltage=100 V  n_fail_on_voltage=1  max_permissible_current=1 A  t_fail_on_current=1 s  iL1_specify=off  iL1_priority=High  iL1=0 A  iL1_nominal_specify=off  iL1_nominal_unit=A  iL1_nominal_value=1  iL2_specify=off  iL2_priority=High  iL2=0 A  iL2_nominal_specify=off  iL2_nominal_unit=A  iL2_nominal_value=1  faulted_specify=off  faulted_priority=None  faulted=0
      settings: InternalSimscapePortConfiguration="{\"Bottom\":[],\"Left\":[{\"id\":\"p1\",\"label\":\"1+\",\"type\":\"foundation.electrical.electrical\"},{\"id\":\"n1\",\"label\":\"1-\",\"type\":\"foundation.electrical.electrical\"}],\"Right\":[{\"id\":\"p2\",\"label\":\"2+\",\"type\":\"foundation.electrical.electrical\"},{\"id\":\"n2\",\"label\":\"2-\",\"type\":\"foundation.electrical.electrical\"}],\"Top\":[]}"
  Offset3 : ee_lib/Sources/Current Source  dc_current=id_l_A*(1-S_a_l) A  ac_current=0 A  ac_shift=0 rad  ac_frequency=0 Hz  noise_mode=0  PSD=0 A^2/Hz  sample_time=1e-3 s  repeatability=1  user_seed=0  auto_seed=3287869569  i_specify=off  i_priority=None  i=0 A  i_nominal_specify=off  i_nominal_unit=A  i_nominal_value=1  v_specify=off  v_priority=None  v=0 V  v_nominal_specify=off  v_nominal_unit=V  v_nominal_value=1
  Offset4 : ee_lib/Sources/Current Source  dc_current=id_l_A*S_a_l A  ac_current=0 A  ac_shift=0 rad  ac_frequency=0 Hz  noise_mode=0  PSD=0 A^2/Hz  sample_time=1e-3 s  repeatability=1  user_seed=0  auto_seed=3415357569  i_specify=off  i_priority=None  i=0 A  i_nominal_specify=off  i_nominal_unit=A  i_nominal_value=1  v_specify=off  v_priority=None  v=0 V  v_nominal_specify=off  v_nominal_unit=V  v_nominal_value=1
  PS-Simulink Converter{,1,3,5} (4 alike) : nesl_utility/PS-Simulink Converter  PhysicalDomain=network_engine_domain  SubClassName=ps_output  LeftPortType=input  RightPortType=output  PseudoPeriodic=off  Frequencies=[]  VectorFormat=inherit  Unit=inherit  AffineConversion=off
  Scope : Scope
  Scope1 : Scope
  Storage : fl_lib/Electrical/Electrical Elements/Capacitor  c=C_g F  r=0 Ohm  g=0 1/Ohm  i_specify=off  i_priority=None  i=0 A  i_nominal_specify=off  i_nominal_unit=A  i_nominal_value=1  v_specify=off  v_priority=None  v=0 V  v_nominal_specify=off  v_nominal_unit=V  v_nominal_value=1  vc_specify=off  vc_priority=High  vc=0 V  vc_nominal_specify=off  vc_nominal_unit=V  vc_nominal_value=1
  Storage1 : fl_lib/Electrical/Electrical Elements/Capacitor  c=C_g F  r=0 Ohm  g=0 1/Ohm  i_specify=off  i_priority=None  i=0 A  i_nominal_specify=off  i_nominal_unit=A  i_nominal_value=1  v_specify=off  v_priority=None  v=0 V  v_nominal_specify=off  v_nominal_unit=V  v_nominal_value=1  vc_specify=off  vc_priority=High  vc=0 V  vc_nominal_specify=off  vc_nominal_unit=V  vc_nominal_value=1
  "i+ " : PMIOPort  Tag=PMCPort  Side=Left
  i+ 1 : PMIOPort  Tag=PMCPort  Port=2  Side=Left
  i- : PMIOPort  Tag=PMCPort  Port=3  Side=Left
  i-1 : PMIOPort  Tag=PMCPort  Port=4  Side=Left
  Out2 : Outport
  Out5 : Outport  Port=2
  wires:
  PS-Simulink Converter3/1 -> Scope1/1
  PS-Simulink Converter5/1 -> Demand comparison/2, Out5/1  "Green"
  PS-Simulink Converter/1 -> Scope/1
  PS-Simulink Converter1/1 -> Out2/1, Demand comparison/1, Gr/1  "Blue etc"
  connections:
  Current Sensor/LConn1 -- L= H2 R= Ammonia/LConn2 -- Offset3/RConn1 -- Current Sensor1/RConn2
  Current Sensor2/LConn1 -- Current Sensor3/RConn2 -- L= H2 R= Ammonia/RConn2 -- Offset4/RConn1
  L= H2 R= Ammonia/LConn1 -- Storage/LConn1 -- i-/RConn1 -- Offset3/LConn1
  L= H2 R= Ammonia/RConn1 -- Storage1/LConn1 -- i-1/RConn1 -- Offset4/LConn1
  Storage1/RConn1 -- Current Sensor2/RConn2
  PS-Simulink Converter3/LConn1 -- Current Sensor2/RConn1
  Current Sensor3/RConn1 -- PS-Simulink Converter5/LConn1
  Current Sensor1/RConn1 -- PS-Simulink Converter1/LConn1
  Storage/RConn1 -- Current Sensor/RConn2
  Current Sensor1/LConn1 -- "i+ "/RConn1
  PS-Simulink Converter/LConn1 -- Current Sensor/RConn1
  Current Sensor3/LConn1 -- i+ 1/RConn1
